simulink model "TxCAN3"  (R2014a)
settings: Solver=ode45  StartTime=0.0  StopTime=10.0  RelTol=1e-3
libraries: simulink x26
settings Model: Creator=10226  LastModifiedBy=10226

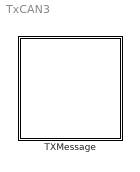
== system TxCAN3 ==
  TXMessage : Subsystem

== system TxCAN3/TXMessage ==
  VCU_AccPedalFault : Ground
  VCU_BMSEmergencyCmd : Ground
  VCU_BMSMainRelayCmd : Ground
  VCU_BrakePedalSts : Ground
  VCU_BrakePedalValue_Reserved : Ground
  VCU_CheckSum : Ground
  VCU_DCDCEnableCmd : Ground
  VCU_DrvControlMode : Ground
  VCU_DrvRequesSpeed : Ground
  VCU_DrvRequestTorque : Ground
  VCU_EA : Subsystem
  VCU_EA_Ter : Terminator
  VCU_ESPTorqReqAvailability : Ground
  VCU_GearLevelPosSts : Ground
  VCU_ParkingReqToEPB : Ground
  VCU_RollingCounter : Ground
  VCU_VehicleSts : Ground
  VCU_Vehicle_Warning : Ground
  wires:
  VCU_ParkingReqToEPB/1 -> VCU_EA/1(VCU_ParkingReqToEPB_in)
  VCU_ESPTorqReqAvailability/1 -> VCU_EA/2(VCU_ESPTorqReqAvailability_in)
  VCU_AccPedalFault/1 -> VCU_EA/3(VCU_AccPedalFault_in)
  VCU_BrakePedalValue_Reserved/1 -> VCU_EA/4(VCU_BrakePedalValue_Reserved_in)
  VCU_CheckSum/1 -> VCU_EA/5(VCU_CheckSum_in)
  VCU_RollingCounter/1 -> VCU_EA/6(VCU_RollingCounter_in)
  VCU_BrakePedalSts/1 -> VCU_EA/7(VCU_BrakePedalSts_in)
  VCU_DCDCEnableCmd/1 -> VCU_EA/8(VCU_DCDCEnableCmd_in)
  VCU_BMSEmergencyCmd/1 -> VCU_EA/9(VCU_BMSEmergencyCmd_in)
  VCU_BMSMainRelayCmd/1 -> VCU_EA/10(VCU_BMSMainRelayCmd_in)
  VCU_GearLevelPosSts/1 -> VCU_EA/11(VCU_GearLevelPosSts_in)
  VCU_VehicleSts/1 -> VCU_EA/12(VCU_VehicleSts_in)
  VCU_Vehicle_Warning/1 -> VCU_EA/13(VCU_Vehicle_Warning_in)
  VCU_DrvControlMode/1 -> VCU_EA/14(VCU_DrvControlMode_in)
  VCU_DrvRequestTorque/1 -> VCU_EA/15(VCU_DrvRequestTorque_in)
  VCU_DrvRequesSpeed/1 -> VCU_EA/16(VCU_DrvRequesSpeed_in)
  VCU_EA/1(output) -> VCU_EA_Ter/1

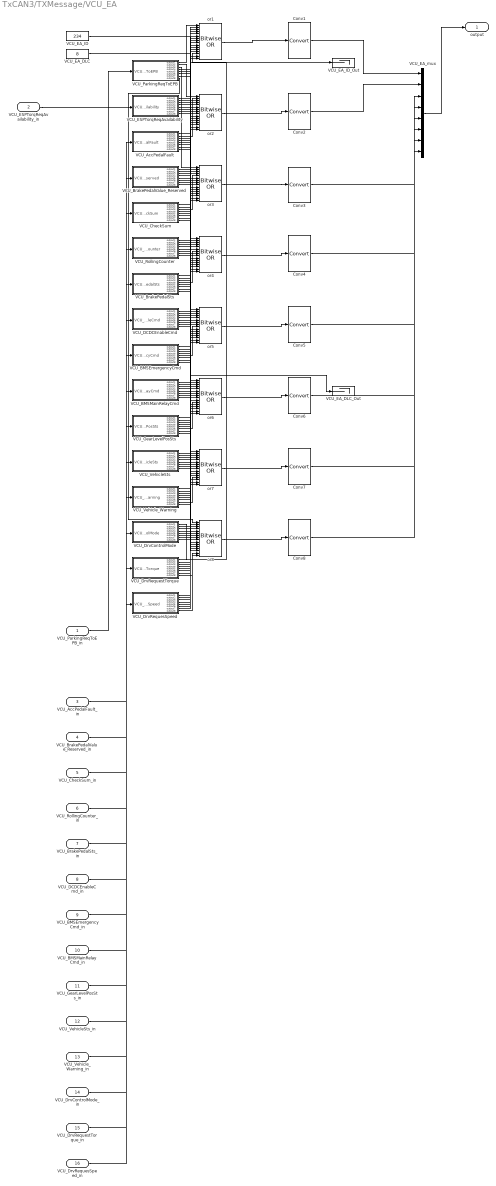
== system TxCAN3/TXMessage/VCU_EA ==
  VCU_ParkingReqToEPB_in : Inport
  VCU_ESPTorqReqAvailability_in : Inport  Port=2
  VCU_AccPedalFault_in : Inport  Port=3
  VCU_BrakePedalValue_Reserved_in : Inport  Port=4
  VCU_CheckSum_in : Inport  Port=5
  VCU_RollingCounter_in : Inport  Port=6
  VCU_BrakePedalSts_in : Inport  Port=7
  VCU_DCDCEnableCmd_in : Inport  Port=8
  VCU_BMSEmergencyCmd_in : Inport  Port=9
  VCU_BMSMainRelayCmd_in : Inport  Port=10
  VCU_GearLevelPosSts_in : Inport  Port=11
  VCU_VehicleSts_in : Inport  Port=12
  VCU_Vehicle_Warning_in : Inport  Port=13
  VCU_DrvControlMode_in : Inport  Port=14
  VCU_DrvRequestTorque_in : Inport  Port=15
  VCU_DrvRequesSpeed_in : Inport  Port=16
  Conv{1..8} (8 alike) : DataTypeConversion
  VCU_AccPedalFault : Subsystem
  VCU_BMSEmergencyCmd : Subsystem
  VCU_BMSMainRelayCmd : Subsystem
  VCU_BrakePedalSts : Subsystem
  VCU_BrakePedalValue_Reserved : Subsystem
  VCU_CheckSum : Subsystem
  VCU_DCDCEnableCmd : Subsystem
  VCU_DrvControlMode : Subsystem
  VCU_DrvRequesSpeed : Subsystem
  VCU_DrvRequestTorque : Subsystem
  VCU_EA_DLC : Constant  Value=8  OutDataTypeStr=uint8
  VCU_EA_DLC_Out : Terminator
  VCU_EA_ID : Constant  Value=234  OutDataTypeStr=single
  VCU_EA_ID_Out : Terminator
  VCU_EA_mux : Mux  Inputs=8
  VCU_ESPTorqReqAvailability : Subsystem
  VCU_GearLevelPosSts : Subsystem
  VCU_ParkingReqToEPB : Subsystem
  VCU_RollingCounter : Subsystem
  VCU_VehicleSts : Subsystem
  VCU_Vehicle_Warning : Subsystem
  or{1..8} (8 alike) : simulink/Logic and Bit Operations/Bitwise Operator  logicop=OR  UseBitMask=off  NumInputPorts=16  BitMask=bin2dec('11011001')  BitMaskRealWorld=Stored Integer
  output : Outport
  wires:
  VCU_EA_mux/1 -> output/1
  VCU_ParkingReqToEPB/1(output1) -> or1/1
  VCU_ParkingReqToEPB/2(output2) -> or2/1
  VCU_ParkingReqToEPB/3(output3) -> or3/1
  VCU_ParkingReqToEPB/4(output4) -> or4/1
  VCU_ParkingReqToEPB/5(output5) -> or5/1
  VCU_ParkingReqToEPB/6(output6) -> or6/1
  VCU_ParkingReqToEPB/7(output7) -> or7/1
  VCU_ParkingReqToEPB/8(output8) -> or8/1
  VCU_ESPTorqReqAvailability/1(output1) -> or1/2
  VCU_ESPTorqReqAvailability/2(output2) -> or2/2
  VCU_ESPTorqReqAvailability/3(output3) -> or3/2
  VCU_ESPTorqReqAvailability/4(output4) -> or4/2
  VCU_ESPTorqReqAvailability/5(output5) -> or5/2
  VCU_ESPTorqReqAvailability/6(output6) -> or6/2
  VCU_ESPTorqReqAvailability/7(output7) -> or7/2
  VCU_ESPTorqReqAvailability/8(output8) -> or8/2
  VCU_AccPedalFault/1(output1) -> or1/3
  VCU_AccPedalFault/2(output2) -> or2/3
  VCU_AccPedalFault/3(output3) -> or3/3
  VCU_AccPedalFault/4(output4) -> or4/3
  VCU_AccPedalFault/5(output5) -> or5/3
  VCU_AccPedalFault/6(output6) -> or6/3
  VCU_AccPedalFault/7(output7) -> or7/3
  VCU_AccPedalFault/8(output8) -> or8/3
  VCU_BrakePedalValue_Reserved/1(output1) -> or1/4
  VCU_BrakePedalValue_Reserved/2(output2) -> or2/4
  VCU_BrakePedalValue_Reserved/3(output3) -> or3/4
  VCU_BrakePedalValue_Reserved/4(output4) -> or4/4
  VCU_BrakePedalValue_Reserved/5(output5) -> or5/4
  VCU_BrakePedalValue_Reserved/6(output6) -> or6/4
  VCU_BrakePedalValue_Reserved/7(output7) -> or7/4
  VCU_BrakePedalValue_Reserved/8(output8) -> or8/4
  VCU_CheckSum/1(output1) -> or1/5
  VCU_CheckSum/2(output2) -> or2/5
  VCU_CheckSum/3(output3) -> or3/5
  VCU_CheckSum/4(output4) -> or4/5
  VCU_CheckSum/5(output5) -> or5/5
  VCU_CheckSum/6(output6) -> or6/5
  VCU_CheckSum/7(output7) -> or7/5
  VCU_CheckSum/8(output8) -> or8/5
  VCU_RollingCounter/1(output1) -> or1/6
  VCU_RollingCounter/2(output2) -> or2/6
  VCU_RollingCounter/3(output3) -> or3/6
  VCU_RollingCounter/4(output4) -> or4/6
  VCU_RollingCounter/5(output5) -> or5/6
  VCU_RollingCounter/6(output6) -> or6/6
  VCU_RollingCounter/7(output7) -> or7/6
  VCU_RollingCounter/8(output8) -> or8/6
  VCU_BrakePedalSts/1(output1) -> or1/7
  VCU_BrakePedalSts/2(output2) -> or2/7
  VCU_BrakePedalSts/3(output3) -> or3/7
  VCU_BrakePedalSts/4(output4) -> or4/7
  VCU_BrakePedalSts/5(output5) -> or5/7
  VCU_BrakePedalSts/6(output6) -> or6/7
  VCU_BrakePedalSts/7(output7) -> or7/7
  VCU_BrakePedalSts/8(output8) -> or8/7
  VCU_DCDCEnableCmd/1(output1) -> or1/8
  VCU_DCDCEnableCmd/2(output2) -> or2/8
  VCU_DCDCEnableCmd/3(output3) -> or3/8
  VCU_DCDCEnableCmd/4(output4) -> or4/8
  VCU_DCDCEnableCmd/5(output5) -> or5/8
  VCU_DCDCEnableCmd/6(output6) -> or6/8
  VCU_DCDCEnableCmd/7(output7) -> or7/8
  VCU_DCDCEnableCmd/8(output8) -> or8/8
  VCU_BMSEmergencyCmd/1(output1) -> or1/9
  VCU_BMSEmergencyCmd/2(output2) -> or2/9
  VCU_BMSEmergencyCmd/3(output3) -> or3/9
  VCU_BMSEmergencyCmd/4(output4) -> or4/9
  VCU_BMSEmergencyCmd/5(output5) -> or5/9
  VCU_BMSEmergencyCmd/6(output6) -> or6/9
  VCU_BMSEmergencyCmd/7(output7) -> or7/9
  VCU_BMSEmergencyCmd/8(output8) -> or8/9
  VCU_BMSMainRelayCmd/1(output1) -> or1/10
  VCU_BMSMainRelayCmd/2(output2) -> or2/10
  VCU_BMSMainRelayCmd/3(output3) -> or3/10
  VCU_BMSMainRelayCmd/4(output4) -> or4/10
  VCU_BMSMainRelayCmd/5(output5) -> or5/10
  VCU_BMSMainRelayCmd/6(output6) -> or6/10
  VCU_BMSMainRelayCmd/7(output7) -> or7/10
  VCU_BMSMainRelayCmd/8(output8) -> or8/10
  VCU_GearLevelPosSts/1(output1) -> or1/11
  VCU_GearLevelPosSts/2(output2) -> or2/11
  VCU_GearLevelPosSts/3(output3) -> or3/11
  VCU_GearLevelPosSts/4(output4) -> or4/11
  VCU_GearLevelPosSts/5(output5) -> or5/11
  VCU_GearLevelPosSts/6(output6) -> or6/11
  VCU_GearLevelPosSts/7(output7) -> or7/11
  VCU_GearLevelPosSts/8(output8) -> or8/11
  VCU_VehicleSts/1(output1) -> or1/12
  VCU_VehicleSts/2(output2) -> or2/12
  VCU_VehicleSts/3(output3) -> or3/12
  VCU_VehicleSts/4(output4) -> or4/12
  VCU_VehicleSts/5(output5) -> or5/12
  VCU_VehicleSts/6(output6) -> or6/12
  VCU_VehicleSts/7(output7) -> or7/12
  VCU_VehicleSts/8(output8) -> or8/12
  VCU_Vehicle_Warning/1(output1) -> or1/13
  VCU_Vehicle_Warning/2(output2) -> or2/13
  VCU_Vehicle_Warning/3(output3) -> or3/13
  VCU_Vehicle_Warning/4(output4) -> or4/13
  VCU_Vehicle_Warning/5(output5) -> or5/13
  VCU_Vehicle_Warning/6(output6) -> or6/13
  VCU_Vehicle_Warning/7(output7) -> or7/13
  VCU_Vehicle_Warning/8(output8) -> or8/13
  VCU_DrvControlMode/1(output1) -> or1/14
  VCU_DrvControlMode/2(output2) -> or2/14
  VCU_DrvControlMode/3(output3) -> or3/14
  VCU_DrvControlMode/4(output4) -> or4/14
  VCU_DrvControlMode/5(output5) -> or5/14
  VCU_DrvControlMode/6(output6) -> or6/14
  VCU_DrvControlMode/7(output7) -> or7/14
  VCU_DrvControlMode/8(output8) -> or8/14
  VCU_DrvRequestTorque/1(output1) -> or1/15
  VCU_DrvRequestTorque/2(output2) -> or2/15
  VCU_DrvRequestTorque/3(output3) -> or3/15
  VCU_DrvRequestTorque/4(output4) -> or4/15
  VCU_DrvRequestTorque/5(output5) -> or5/15
  VCU_DrvRequestTorque/6(output6) -> or6/15
  VCU_DrvRequestTorque/7(output7) -> or7/15
  VCU_DrvRequestTorque/8(output8) -> or8/15
  VCU_DrvRequesSpeed/1(output1) -> or1/16
  VCU_DrvRequesSpeed/2(output2) -> or2/16
  VCU_DrvRequesSpeed/3(output3) -> or3/16
  VCU_DrvRequesSpeed/4(output4) -> or4/16
  VCU_DrvRequesSpeed/5(output5) -> or5/16
  VCU_DrvRequesSpeed/6(output6) -> or6/16
  VCU_DrvRequesSpeed/7(output7) -> or7/16
  VCU_DrvRequesSpeed/8(output8) -> or8/16
  or1/1 -> Conv1/1
  Conv1/1 -> VCU_EA_mux/1
  or2/1 -> Conv2/1
  Conv2/1 -> VCU_EA_mux/2
  or3/1 -> Conv3/1
  Conv3/1 -> VCU_EA_mux/3
  or4/1 -> Conv4/1
  Conv4/1 -> VCU_EA_mux/4
  or5/1 -> Conv5/1
  Conv5/1 -> VCU_EA_mux/5
  or6/1 -> Conv6/1
  Conv6/1 -> VCU_EA_mux/6
  or7/1 -> Conv7/1
  Conv7/1 -> VCU_EA_mux/7
  or8/1 -> Conv8/1
  Conv8/1 -> VCU_EA_mux/8
  VCU_EA_ID/1 -> VCU_EA_ID_Out/1
  VCU_EA_DLC/1 -> VCU_EA_DLC_Out/1
  VCU_ParkingReqToEPB_in/1 -> VCU_ParkingReqToEPB/1(VCU_ParkingReqToEPB)
  VCU_ESPTorqReqAvailability_in/1 -> VCU_ESPTorqReqAvailability/1(VCU_ESPTorqReqAvailability)
  VCU_AccPedalFault_in/1 -> VCU_AccPedalFault/1(VCU_AccPedalFault)
  VCU_BrakePedalValue_Reserved_in/1 -> VCU_BrakePedalValue_Reserved/1(VCU_BrakePedalValue_Reserved)
  VCU_CheckSum_in/1 -> VCU_CheckSum/1(VCU_CheckSum)
  VCU_RollingCounter_in/1 -> VCU_RollingCounter/1(VCU_RollingCounter)
  VCU_BrakePedalSts_in/1 -> VCU_BrakePedalSts/1(VCU_BrakePedalSts)
  VCU_DCDCEnableCmd_in/1 -> VCU_DCDCEnableCmd/1(VCU_DCDCEnableCmd)
  VCU_BMSEmergencyCmd_in/1 -> VCU_BMSEmergencyCmd/1(VCU_BMSEmergencyCmd)
  VCU_BMSMainRelayCmd_in/1 -> VCU_BMSMainRelayCmd/1(VCU_BMSMainRelayCmd)
  VCU_GearLevelPosSts_in/1 -> VCU_GearLevelPosSts/1(VCU_GearLevelPosSts)
  VCU_VehicleSts_in/1 -> VCU_VehicleSts/1(VCU_VehicleSts)
  VCU_Vehicle_Warning_in/1 -> VCU_Vehicle_Warning/1(VCU_Vehicle_Warning)
  VCU_DrvControlMode_in/1 -> VCU_DrvControlMode/1(VCU_DrvControlMode)
  VCU_DrvRequestTorque_in/1 -> VCU_DrvRequestTorque/1(VCU_DrvRequestTorque)
  VCU_DrvRequesSpeed_in/1 -> VCU_DrvRequesSpeed/1(VCU_DrvRequesSpeed)

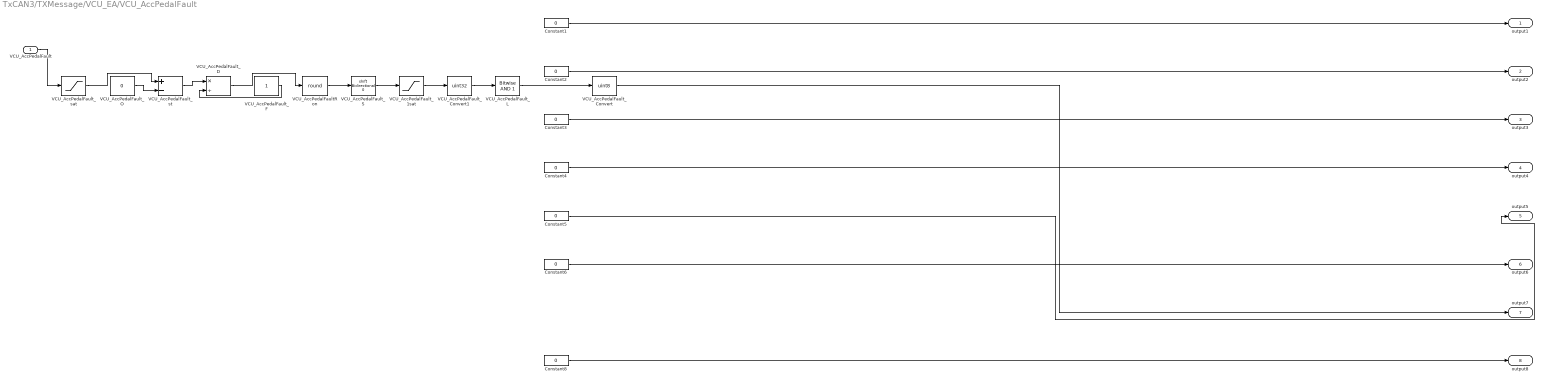
== system TxCAN3/TXMessage/VCU_EA/VCU_AccPedalFault ==
  VCU_AccPedalFault : Inport
  Constant{1..6,8} (7 alike) : Constant  Value=0  OutDataTypeStr=uint8
  VCU_AccPedalFaultRon : Rounding  Operator=round
  VCU_AccPedalFault_1sat : Saturate  UpperLimit=1  LowerLimit=0
  VCU_AccPedalFault_Convert : DataTypeConversion  OutDataTypeStr=uint8
  VCU_AccPedalFault_Convert1 : DataTypeConversion  OutDataTypeStr=uint32
  VCU_AccPedalFault_D : Product  Inputs=*/
  VCU_AccPedalFault_F : Constant  OutDataTypeStr=single
  VCU_AccPedalFault_L : simulink/Logic and Bit Operations/Bitwise Operator  logicop=AND  UseBitMask=on  BitMask=1  BitMaskRealWorld=Stored Integer
  VCU_AccPedalFault_O : Constant  Value=0  OutDataTypeStr=single
  VCU_AccPedalFault_S : ArithShift
  VCU_AccPedalFault_sat : Saturate  UpperLimit=1  LowerLimit=0
  VCU_AccPedalFault_st : Sum  Inputs=+-
  output1 : Outport
  output2 : Outport  Port=2
  output3 : Outport  Port=3
  output4 : Outport  Port=4
  output5 : Outport  Port=5
  output6 : Outport  Port=6
  output7 : Outport  Port=7
  output8 : Outport  Port=8
  wires:
  VCU_AccPedalFault/1 -> VCU_AccPedalFault_sat/1
  VCU_AccPedalFault_sat/1 -> VCU_AccPedalFault_st/1
  VCU_AccPedalFault_O/1 -> VCU_AccPedalFault_st/2
  VCU_AccPedalFault_st/1 -> VCU_AccPedalFault_D/1
  VCU_AccPedalFault_F/1 -> VCU_AccPedalFault_D/2
  VCU_AccPedalFault_D/1 -> VCU_AccPedalFaultRon/1
  VCU_AccPedalFaultRon/1 -> VCU_AccPedalFault_S/1
  VCU_AccPedalFault_S/1 -> VCU_AccPedalFault_1sat/1
  VCU_AccPedalFault_1sat/1 -> VCU_AccPedalFault_Convert1/1
  VCU_AccPedalFault_Convert1/1 -> VCU_AccPedalFault_L/1
  VCU_AccPedalFault_L/1 -> VCU_AccPedalFault_Convert/1
  VCU_AccPedalFault_Convert/1 -> output7/1
  Constant1/1 -> output1/1
  Constant2/1 -> output2/1
  Constant3/1 -> output3/1
  Constant4/1 -> output4/1
  Constant5/1 -> output5/1
  Constant6/1 -> output6/1
  Constant8/1 -> output8/1

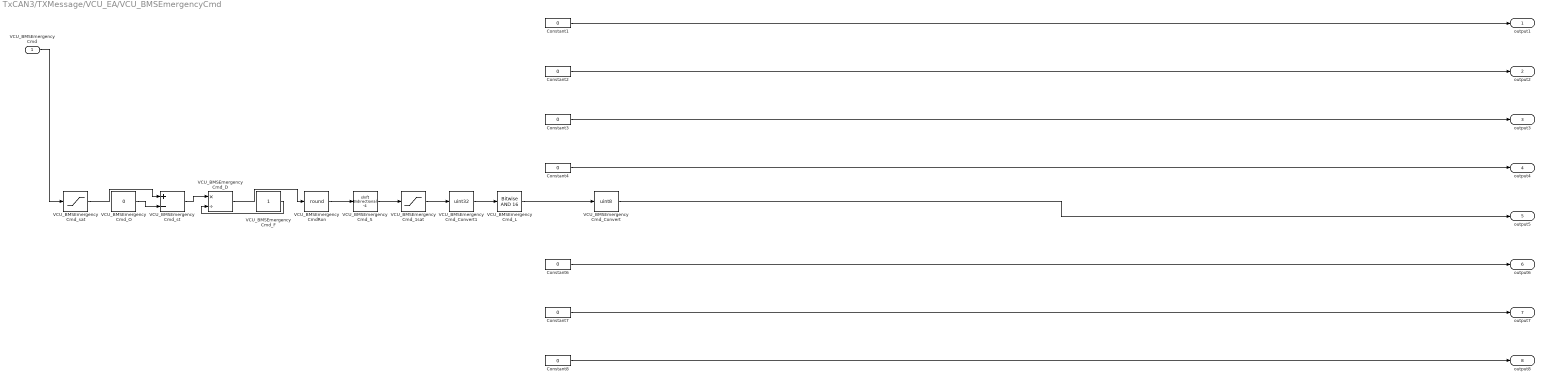
== system TxCAN3/TXMessage/VCU_EA/VCU_BMSEmergencyCmd ==
  VCU_BMSEmergencyCmd : Inport
  Constant{1..4,6..8} (7 alike) : Constant  Value=0  OutDataTypeStr=uint8
  VCU_BMSEmergencyCmdRon : Rounding  Operator=round
  VCU_BMSEmergencyCmd_1sat : Saturate  UpperLimit=16  LowerLimit=0
  VCU_BMSEmergencyCmd_Convert : DataTypeConversion  OutDataTypeStr=uint8
  VCU_BMSEmergencyCmd_Convert1 : DataTypeConversion  OutDataTypeStr=uint32
  VCU_BMSEmergencyCmd_D : Product  Inputs=*/
  VCU_BMSEmergencyCmd_F : Constant  OutDataTypeStr=single
  VCU_BMSEmergencyCmd_L : simulink/Logic and Bit Operations/Bitwise Operator  logicop=AND  UseBitMask=on  BitMask=16  BitMaskRealWorld=Stored Integer
  VCU_BMSEmergencyCmd_O : Constant  Value=0  OutDataTypeStr=single
  VCU_BMSEmergencyCmd_S : ArithShift  BitShiftNumber=-4
  VCU_BMSEmergencyCmd_sat : Saturate  UpperLimit=1  LowerLimit=0
  VCU_BMSEmergencyCmd_st : Sum  Inputs=+-
  output1 : Outport
  output2 : Outport  Port=2
  output3 : Outport  Port=3
  output4 : Outport  Port=4
  output5 : Outport  Port=5
  output6 : Outport  Port=6
  output7 : Outport  Port=7
  output8 : Outport  Port=8
  wires:
  VCU_BMSEmergencyCmd/1 -> VCU_BMSEmergencyCmd_sat/1
  VCU_BMSEmergencyCmd_sat/1 -> VCU_BMSEmergencyCmd_st/1
  VCU_BMSEmergencyCmd_O/1 -> VCU_BMSEmergencyCmd_st/2
  VCU_BMSEmergencyCmd_st/1 -> VCU_BMSEmergencyCmd_D/1
  VCU_BMSEmergencyCmd_F/1 -> VCU_BMSEmergencyCmd_D/2
  VCU_BMSEmergencyCmd_D/1 -> VCU_BMSEmergencyCmdRon/1
  VCU_BMSEmergencyCmdRon/1 -> VCU_BMSEmergencyCmd_S/1
  VCU_BMSEmergencyCmd_S/1 -> VCU_BMSEmergencyCmd_1sat/1
  VCU_BMSEmergencyCmd_1sat/1 -> VCU_BMSEmergencyCmd_Convert1/1
  VCU_BMSEmergencyCmd_Convert1/1 -> VCU_BMSEmergencyCmd_L/1
  VCU_BMSEmergencyCmd_L/1 -> VCU_BMSEmergencyCmd_Convert/1
  VCU_BMSEmergencyCmd_Convert/1 -> output5/1
  Constant1/1 -> output1/1
  Constant2/1 -> output2/1
  Constant3/1 -> output3/1
  Constant4/1 -> output4/1
  Constant6/1 -> output6/1
  Constant7/1 -> output7/1
  Constant8/1 -> output8/1

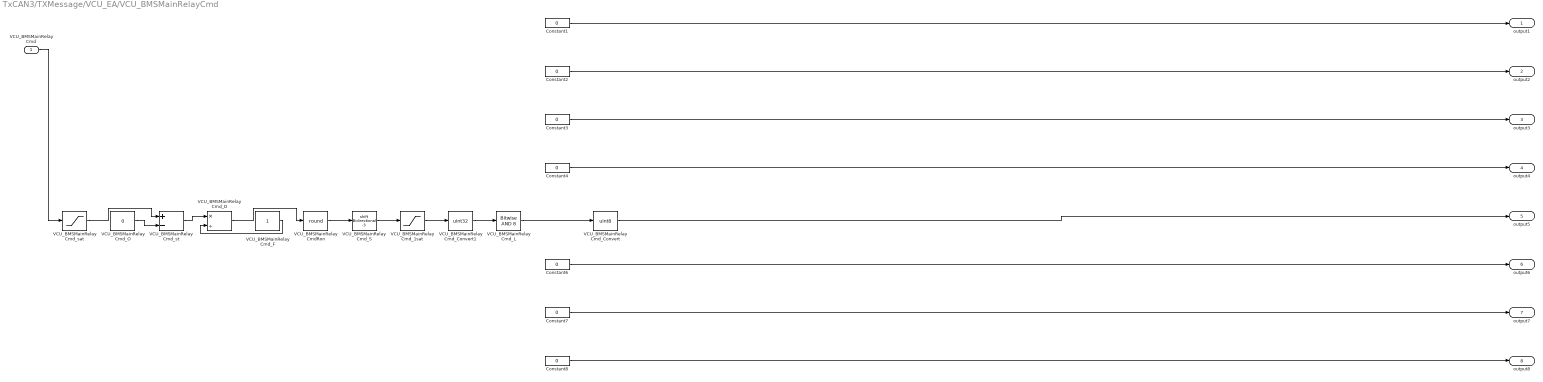
== system TxCAN3/TXMessage/VCU_EA/VCU_BMSMainRelayCmd ==
  VCU_BMSMainRelayCmd : Inport
  Constant{1..4,6..8} (7 alike) : Constant  Value=0  OutDataTypeStr=uint8
  VCU_BMSMainRelayCmdRon : Rounding  Operator=round
  VCU_BMSMainRelayCmd_1sat : Saturate  UpperLimit=8  LowerLimit=0
  VCU_BMSMainRelayCmd_Convert : DataTypeConversion  OutDataTypeStr=uint8
  VCU_BMSMainRelayCmd_Convert1 : DataTypeConversion  OutDataTypeStr=uint32
  VCU_BMSMainRelayCmd_D : Product  Inputs=*/
  VCU_BMSMainRelayCmd_F : Constant  OutDataTypeStr=single
  VCU_BMSMainRelayCmd_L : simulink/Logic and Bit Operations/Bitwise Operator  logicop=AND  UseBitMask=on  BitMask=8  BitMaskRealWorld=Stored Integer
  VCU_BMSMainRelayCmd_O : Constant  Value=0  OutDataTypeStr=single
  VCU_BMSMainRelayCmd_S : ArithShift  BitShiftNumber=-3
  VCU_BMSMainRelayCmd_sat : Saturate  UpperLimit=1  LowerLimit=0
  VCU_BMSMainRelayCmd_st : Sum  Inputs=+-
  output1 : Outport
  output2 : Outport  Port=2
  output3 : Outport  Port=3
  output4 : Outport  Port=4
  output5 : Outport  Port=5
  output6 : Outport  Port=6
  output7 : Outport  Port=7
  output8 : Outport  Port=8
  wires:
  VCU_BMSMainRelayCmd/1 -> VCU_BMSMainRelayCmd_sat/1
  VCU_BMSMainRelayCmd_sat/1 -> VCU_BMSMainRelayCmd_st/1
  VCU_BMSMainRelayCmd_O/1 -> VCU_BMSMainRelayCmd_st/2
  VCU_BMSMainRelayCmd_st/1 -> VCU_BMSMainRelayCmd_D/1
  VCU_BMSMainRelayCmd_F/1 -> VCU_BMSMainRelayCmd_D/2
  VCU_BMSMainRelayCmd_D/1 -> VCU_BMSMainRelayCmdRon/1
  VCU_BMSMainRelayCmdRon/1 -> VCU_BMSMainRelayCmd_S/1
  VCU_BMSMainRelayCmd_S/1 -> VCU_BMSMainRelayCmd_1sat/1
  VCU_BMSMainRelayCmd_1sat/1 -> VCU_BMSMainRelayCmd_Convert1/1
  VCU_BMSMainRelayCmd_Convert1/1 -> VCU_BMSMainRelayCmd_L/1
  VCU_BMSMainRelayCmd_L/1 -> VCU_BMSMainRelayCmd_Convert/1
  VCU_BMSMainRelayCmd_Convert/1 -> output5/1
  Constant1/1 -> output1/1
  Constant2/1 -> output2/1
  Constant3/1 -> output3/1
  Constant4/1 -> output4/1
  Constant6/1 -> output6/1
  Constant7/1 -> output7/1
  Constant8/1 -> output8/1

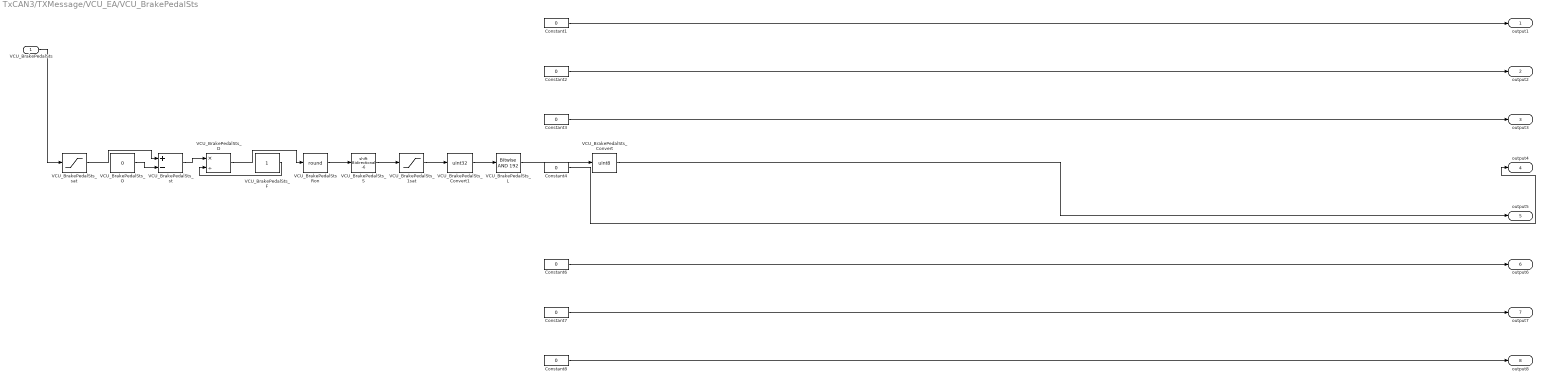
== system TxCAN3/TXMessage/VCU_EA/VCU_BrakePedalSts ==
  VCU_BrakePedalSts : Inport
  Constant{1..4,6..8} (7 alike) : Constant  Value=0  OutDataTypeStr=uint8
  VCU_BrakePedalStsRon : Rounding  Operator=round
  VCU_BrakePedalSts_1sat : Saturate  UpperLimit=192  LowerLimit=0
  VCU_BrakePedalSts_Convert : DataTypeConversion  OutDataTypeStr=uint8
  VCU_BrakePedalSts_Convert1 : DataTypeConversion  OutDataTypeStr=uint32
  VCU_BrakePedalSts_D : Product  Inputs=*/
  VCU_BrakePedalSts_F : Constant  OutDataTypeStr=single
  VCU_BrakePedalSts_L : simulink/Logic and Bit Operations/Bitwise Operator  logicop=AND  UseBitMask=on  BitMask=192  BitMaskRealWorld=Stored Integer
  VCU_BrakePedalSts_O : Constant  Value=0  OutDataTypeStr=single
  VCU_BrakePedalSts_S : ArithShift  BitShiftNumber=-6
  VCU_BrakePedalSts_sat : Saturate  UpperLimit=3  LowerLimit=0
  VCU_BrakePedalSts_st : Sum  Inputs=+-
  output1 : Outport
  output2 : Outport  Port=2
  output3 : Outport  Port=3
  output4 : Outport  Port=4
  output5 : Outport  Port=5
  output6 : Outport  Port=6
  output7 : Outport  Port=7
  output8 : Outport  Port=8
  wires:
  VCU_BrakePedalSts/1 -> VCU_BrakePedalSts_sat/1
  VCU_BrakePedalSts_sat/1 -> VCU_BrakePedalSts_st/1
  VCU_BrakePedalSts_O/1 -> VCU_BrakePedalSts_st/2
  VCU_BrakePedalSts_st/1 -> VCU_BrakePedalSts_D/1
  VCU_BrakePedalSts_F/1 -> VCU_BrakePedalSts_D/2
  VCU_BrakePedalSts_D/1 -> VCU_BrakePedalStsRon/1
  VCU_BrakePedalStsRon/1 -> VCU_BrakePedalSts_S/1
  VCU_BrakePedalSts_S/1 -> VCU_BrakePedalSts_1sat/1
  VCU_BrakePedalSts_1sat/1 -> VCU_BrakePedalSts_Convert1/1
  VCU_BrakePedalSts_Convert1/1 -> VCU_BrakePedalSts_L/1
  VCU_BrakePedalSts_L/1 -> VCU_BrakePedalSts_Convert/1
  VCU_BrakePedalSts_Convert/1 -> output5/1
  Constant1/1 -> output1/1
  Constant2/1 -> output2/1
  Constant3/1 -> output3/1
  Constant4/1 -> output4/1
  Constant6/1 -> output6/1
  Constant7/1 -> output7/1
  Constant8/1 -> output8/1

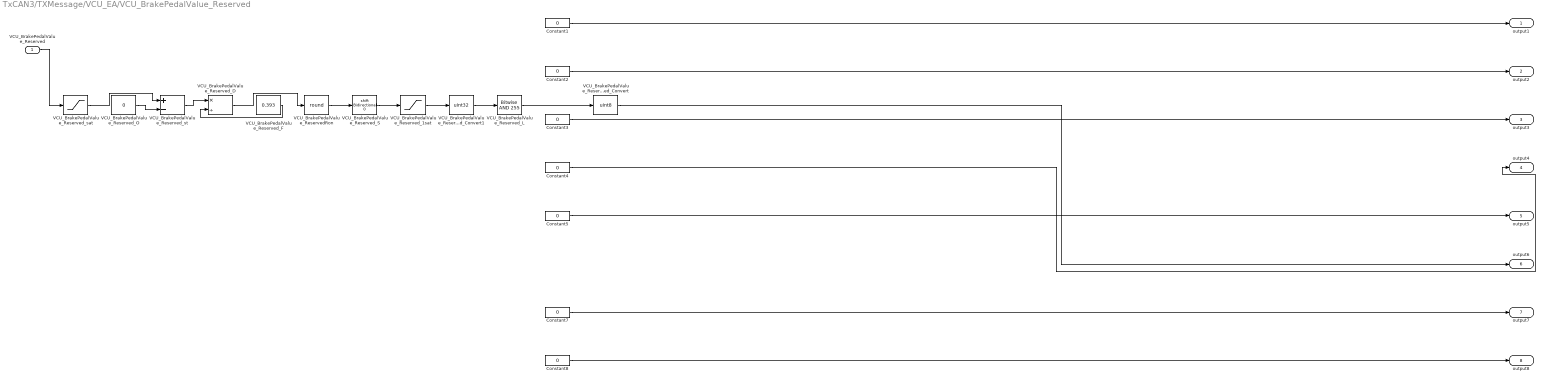
== system TxCAN3/TXMessage/VCU_EA/VCU_BrakePedalValue_Reserved ==
  VCU_BrakePedalValue_Reserved : Inport
  Constant{1..5,7..8} (7 alike) : Constant  Value=0  OutDataTypeStr=uint8
  VCU_BrakePedalValue_ReservedRon : Rounding  Operator=round
  VCU_BrakePedalValue_Reserved_1sat : Saturate  UpperLimit=255  LowerLimit=0
  VCU_BrakePedalValue_Reserved_Convert : DataTypeConversion  OutDataTypeStr=uint8
  VCU_BrakePedalValue_Reserved_Convert1 : DataTypeConversion  OutDataTypeStr=uint32
  VCU_BrakePedalValue_Reserved_D : Product  Inputs=*/
  VCU_BrakePedalValue_Reserved_F : Constant  Value=0.393  OutDataTypeStr=single
  VCU_BrakePedalValue_Reserved_L : simulink/Logic and Bit Operations/Bitwise Operator  logicop=AND  UseBitMask=on  BitMask=255  BitMaskRealWorld=Stored Integer
  VCU_BrakePedalValue_Reserved_O : Constant  Value=0  OutDataTypeStr=single
  VCU_BrakePedalValue_Reserved_S : ArithShift
  VCU_BrakePedalValue_Reserved_sat : Saturate  UpperLimit=100  LowerLimit=0
  VCU_BrakePedalValue_Reserved_st : Sum  Inputs=+-
  output1 : Outport
  output2 : Outport  Port=2
  output3 : Outport  Port=3
  output4 : Outport  Port=4
  output5 : Outport  Port=5
  output6 : Outport  Port=6
  output7 : Outport  Port=7
  output8 : Outport  Port=8
  wires:
  VCU_BrakePedalValue_Reserved/1 -> VCU_BrakePedalValue_Reserved_sat/1
  VCU_BrakePedalValue_Reserved_sat/1 -> VCU_BrakePedalValue_Reserved_st/1
  VCU_BrakePedalValue_Reserved_O/1 -> VCU_BrakePedalValue_Reserved_st/2
  VCU_BrakePedalValue_Reserved_st/1 -> VCU_BrakePedalValue_Reserved_D/1
  VCU_BrakePedalValue_Reserved_F/1 -> VCU_BrakePedalValue_Reserved_D/2
  VCU_BrakePedalValue_Reserved_D/1 -> VCU_BrakePedalValue_ReservedRon/1
  VCU_BrakePedalValue_ReservedRon/1 -> VCU_BrakePedalValue_Reserved_S/1
  VCU_BrakePedalValue_Reserved_S/1 -> VCU_BrakePedalValue_Reserved_1sat/1
  VCU_BrakePedalValue_Reserved_1sat/1 -> VCU_BrakePedalValue_Reserved_Convert1/1
  VCU_BrakePedalValue_Reserved_Convert1/1 -> VCU_BrakePedalValue_Reserved_L/1
  VCU_BrakePedalValue_Reserved_L/1 -> VCU_BrakePedalValue_Reserved_Convert/1
  VCU_BrakePedalValue_Reserved_Convert/1 -> output6/1
  Constant1/1 -> output1/1
  Constant2/1 -> output2/1
  Constant3/1 -> output3/1
  Constant4/1 -> output4/1
  Constant5/1 -> output5/1
  Constant7/1 -> output7/1
  Constant8/1 -> output8/1

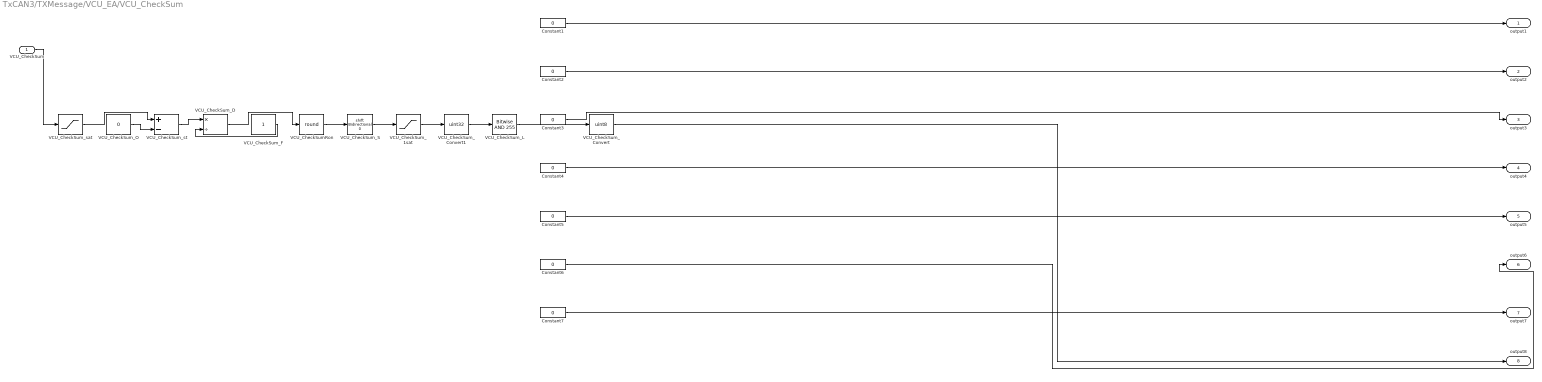
== system TxCAN3/TXMessage/VCU_EA/VCU_CheckSum ==
  VCU_CheckSum : Inport
  Constant{1..7} (7 alike) : Constant  Value=0  OutDataTypeStr=uint8
  VCU_CheckSumRon : Rounding  Operator=round
  VCU_CheckSum_1sat : Saturate  UpperLimit=255  LowerLimit=0
  VCU_CheckSum_Convert : DataTypeConversion  OutDataTypeStr=uint8
  VCU_CheckSum_Convert1 : DataTypeConversion  OutDataTypeStr=uint32
  VCU_CheckSum_D : Product  Inputs=*/
  VCU_CheckSum_F : Constant  OutDataTypeStr=single
  VCU_CheckSum_L : simulink/Logic and Bit Operations/Bitwise Operator  logicop=AND  UseBitMask=on  BitMask=255  BitMaskRealWorld=Stored Integer
  VCU_CheckSum_O : Constant  Value=0  OutDataTypeStr=single
  VCU_CheckSum_S : ArithShift
  VCU_CheckSum_sat : Saturate  UpperLimit=255  LowerLimit=0
  VCU_CheckSum_st : Sum  Inputs=+-
  output1 : Outport
  output2 : Outport  Port=2
  output3 : Outport  Port=3
  output4 : Outport  Port=4
  output5 : Outport  Port=5
  output6 : Outport  Port=6
  output7 : Outport  Port=7
  output8 : Outport  Port=8
  wires:
  VCU_CheckSum/1 -> VCU_CheckSum_sat/1
  VCU_CheckSum_sat/1 -> VCU_CheckSum_st/1
  VCU_CheckSum_O/1 -> VCU_CheckSum_st/2
  VCU_CheckSum_st/1 -> VCU_CheckSum_D/1
  VCU_CheckSum_F/1 -> VCU_CheckSum_D/2
  VCU_CheckSum_D/1 -> VCU_CheckSumRon/1
  VCU_CheckSumRon/1 -> VCU_CheckSum_S/1
  VCU_CheckSum_S/1 -> VCU_CheckSum_1sat/1
  VCU_CheckSum_1sat/1 -> VCU_CheckSum_Convert1/1
  VCU_CheckSum_Convert1/1 -> VCU_CheckSum_L/1
  VCU_CheckSum_L/1 -> VCU_CheckSum_Convert/1
  VCU_CheckSum_Convert/1 -> output8/1
  Constant1/1 -> output1/1
  Constant2/1 -> output2/1
  Constant3/1 -> output3/1
  Constant4/1 -> output4/1
  Constant5/1 -> output5/1
  Constant6/1 -> output6/1
  Constant7/1 -> output7/1

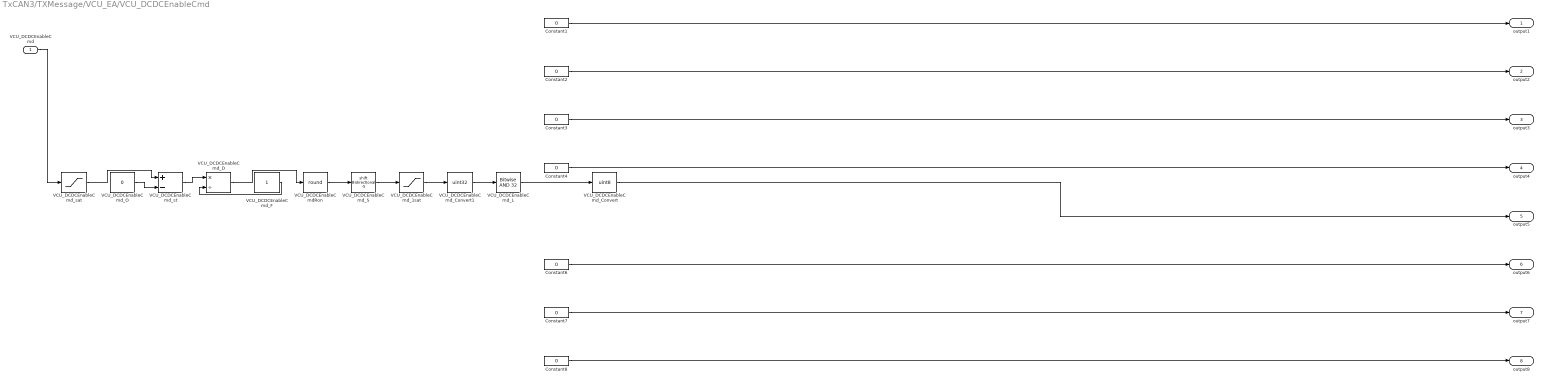
== system TxCAN3/TXMessage/VCU_EA/VCU_DCDCEnableCmd ==
  VCU_DCDCEnableCmd : Inport
  Constant{1..4,6..8} (7 alike) : Constant  Value=0  OutDataTypeStr=uint8
  VCU_DCDCEnableCmdRon : Rounding  Operator=round
  VCU_DCDCEnableCmd_1sat : Saturate  UpperLimit=32  LowerLimit=0
  VCU_DCDCEnableCmd_Convert : DataTypeConversion  OutDataTypeStr=uint8
  VCU_DCDCEnableCmd_Convert1 : DataTypeConversion  OutDataTypeStr=uint32
  VCU_DCDCEnableCmd_D : Product  Inputs=*/
  VCU_DCDCEnableCmd_F : Constant  OutDataTypeStr=single
  VCU_DCDCEnableCmd_L : simulink/Logic and Bit Operations/Bitwise Operator  logicop=AND  UseBitMask=on  BitMask=32  BitMaskRealWorld=Stored Integer
  VCU_DCDCEnableCmd_O : Constant  Value=0  OutDataTypeStr=single
  VCU_DCDCEnableCmd_S : ArithShift  BitShiftNumber=-5
  VCU_DCDCEnableCmd_sat : Saturate  UpperLimit=1  LowerLimit=0
  VCU_DCDCEnableCmd_st : Sum  Inputs=+-
  output1 : Outport
  output2 : Outport  Port=2
  output3 : Outport  Port=3
  output4 : Outport  Port=4
  output5 : Outport  Port=5
  output6 : Outport  Port=6
  output7 : Outport  Port=7
  output8 : Outport  Port=8
  wires:
  VCU_DCDCEnableCmd/1 -> VCU_DCDCEnableCmd_sat/1
  VCU_DCDCEnableCmd_sat/1 -> VCU_DCDCEnableCmd_st/1
  VCU_DCDCEnableCmd_O/1 -> VCU_DCDCEnableCmd_st/2
  VCU_DCDCEnableCmd_st/1 -> VCU_DCDCEnableCmd_D/1
  VCU_DCDCEnableCmd_F/1 -> VCU_DCDCEnableCmd_D/2
  VCU_DCDCEnableCmd_D/1 -> VCU_DCDCEnableCmdRon/1
  VCU_DCDCEnableCmdRon/1 -> VCU_DCDCEnableCmd_S/1
  VCU_DCDCEnableCmd_S/1 -> VCU_DCDCEnableCmd_1sat/1
  VCU_DCDCEnableCmd_1sat/1 -> VCU_DCDCEnableCmd_Convert1/1
  VCU_DCDCEnableCmd_Convert1/1 -> VCU_DCDCEnableCmd_L/1
  VCU_DCDCEnableCmd_L/1 -> VCU_DCDCEnableCmd_Convert/1
  VCU_DCDCEnableCmd_Convert/1 -> output5/1
  Constant1/1 -> output1/1
  Constant2/1 -> output2/1
  Constant3/1 -> output3/1
  Constant4/1 -> output4/1
  Constant6/1 -> output6/1
  Constant7/1 -> output7/1
  Constant8/1 -> output8/1

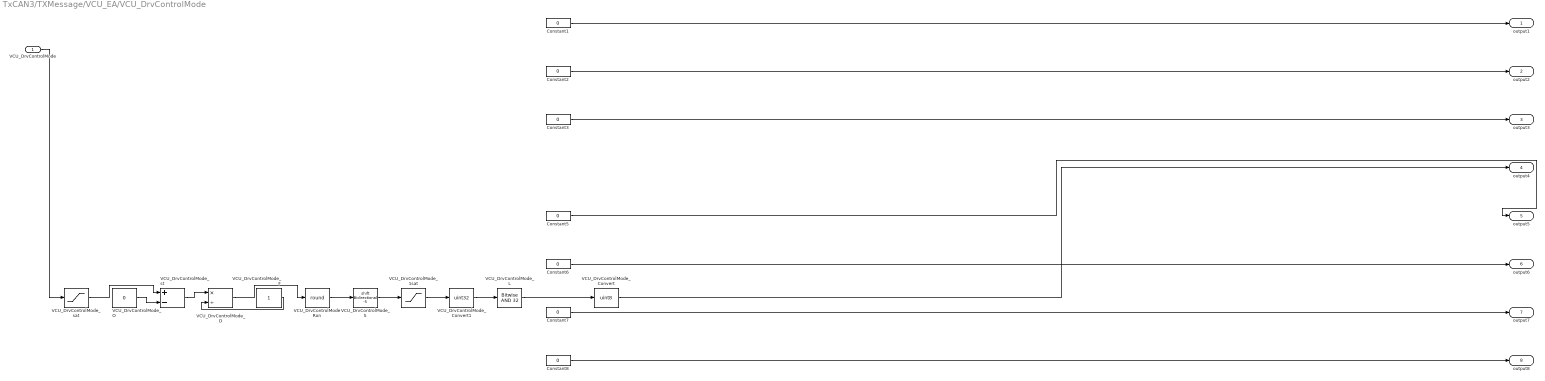
== system TxCAN3/TXMessage/VCU_EA/VCU_DrvControlMode ==
  VCU_DrvControlMode : Inport
  Constant{1..3,5..8} (7 alike) : Constant  Value=0  OutDataTypeStr=uint8
  VCU_DrvControlModeRon : Rounding  Operator=round
  VCU_DrvControlMode_1sat : Saturate  UpperLimit=32  LowerLimit=0
  VCU_DrvControlMode_Convert : DataTypeConversion  OutDataTypeStr=uint8
  VCU_DrvControlMode_Convert1 : DataTypeConversion  OutDataTypeStr=uint32
  VCU_DrvControlMode_D : Product  Inputs=*/
  VCU_DrvControlMode_F : Constant  OutDataTypeStr=single
  VCU_DrvControlMode_L : simulink/Logic and Bit Operations/Bitwise Operator  logicop=AND  UseBitMask=on  BitMask=32  BitMaskRealWorld=Stored Integer
  VCU_DrvControlMode_O : Constant  Value=0  OutDataTypeStr=single
  VCU_DrvControlMode_S : ArithShift  BitShiftNumber=-5
  VCU_DrvControlMode_sat : Saturate  UpperLimit=1  LowerLimit=0
  VCU_DrvControlMode_st : Sum  Inputs=+-
  output1 : Outport
  output2 : Outport  Port=2
  output3 : Outport  Port=3
  output4 : Outport  Port=4
  output5 : Outport  Port=5
  output6 : Outport  Port=6
  output7 : Outport  Port=7
  output8 : Outport  Port=8
  wires:
  VCU_DrvControlMode/1 -> VCU_DrvControlMode_sat/1
  VCU_DrvControlMode_sat/1 -> VCU_DrvControlMode_st/1
  VCU_DrvControlMode_O/1 -> VCU_DrvControlMode_st/2
  VCU_DrvControlMode_st/1 -> VCU_DrvControlMode_D/1
  VCU_DrvControlMode_F/1 -> VCU_DrvControlMode_D/2
  VCU_DrvControlMode_D/1 -> VCU_DrvControlModeRon/1
  VCU_DrvControlModeRon/1 -> VCU_DrvControlMode_S/1
  VCU_DrvControlMode_S/1 -> VCU_DrvControlMode_1sat/1
  VCU_DrvControlMode_1sat/1 -> VCU_DrvControlMode_Convert1/1
  VCU_DrvControlMode_Convert1/1 -> VCU_DrvControlMode_L/1
  VCU_DrvControlMode_L/1 -> VCU_DrvControlMode_Convert/1
  VCU_DrvControlMode_Convert/1 -> output4/1
  Constant1/1 -> output1/1
  Constant2/1 -> output2/1
  Constant3/1 -> output3/1
  Constant5/1 -> output5/1
  Constant6/1 -> output6/1
  Constant7/1 -> output7/1
  Constant8/1 -> output8/1

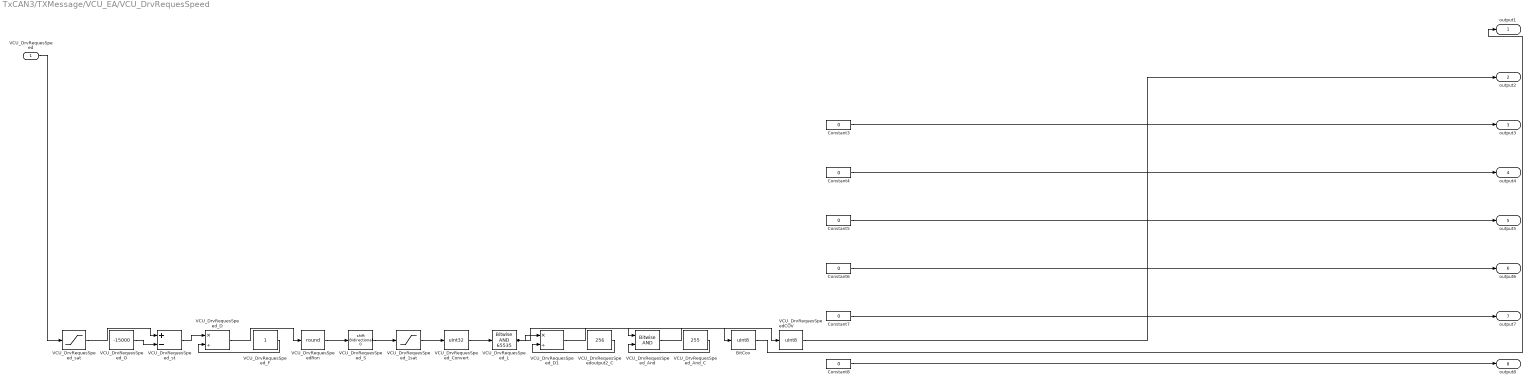
== system TxCAN3/TXMessage/VCU_EA/VCU_DrvRequesSpeed ==
  VCU_DrvRequesSpeed : Inport
  BitCov : DataTypeConversion  OutDataTypeStr=uint8
  Constant{3..8} (6 alike) : Constant  Value=0  OutDataTypeStr=uint8
  VCU_DrvRequesSpeedCOV : DataTypeConversion  OutDataTypeStr=uint8
  VCU_DrvRequesSpeedRon : Rounding  Operator=round
  VCU_DrvRequesSpeed_1sat : Saturate  UpperLimit=65535  LowerLimit=0
  VCU_DrvRequesSpeed_And : simulink/Logic and Bit Operations/Bitwise Operator  logicop=AND  UseBitMask=off  NumInputPorts=2  BitMask=bin2dec('11011001')  BitMaskRealWorld=Stored Integer
  VCU_DrvRequesSpeed_And_C : Constant  Value=255  OutDataTypeStr=uint32
  VCU_DrvRequesSpeed_Convert : DataTypeConversion  OutDataTypeStr=uint32
  VCU_DrvRequesSpeed_D : Product  Inputs=*/
  VCU_DrvRequesSpeed_D1 : Product  Inputs=*/
  VCU_DrvRequesSpeed_F : Constant  OutDataTypeStr=single
  VCU_DrvRequesSpeed_L : simulink/Logic and Bit Operations/Bitwise Operator  logicop=AND  UseBitMask=on  BitMask=65535  BitMaskRealWorld=Stored Integer
  VCU_DrvRequesSpeed_O : Constant  Value=-15000  OutDataTypeStr=single
  VCU_DrvRequesSpeed_S : ArithShift
  VCU_DrvRequesSpeed_sat : Saturate  UpperLimit=15000  LowerLimit=-15000
  VCU_DrvRequesSpeed_st : Sum  Inputs=+-
  VCU_DrvRequesSpeedoutput2_C : Constant  Value=256
  output1 : Outport
  output2 : Outport  Port=2
  output3 : Outport  Port=3
  output4 : Outport  Port=4
  output5 : Outport  Port=5
  output6 : Outport  Port=6
  output7 : Outport  Port=7
  output8 : Outport  Port=8
  wires:
  VCU_DrvRequesSpeed/1 -> VCU_DrvRequesSpeed_sat/1
  VCU_DrvRequesSpeed_sat/1 -> VCU_DrvRequesSpeed_st/1
  VCU_DrvRequesSpeed_O/1 -> VCU_DrvRequesSpeed_st/2
  VCU_DrvRequesSpeed_st/1 -> VCU_DrvRequesSpeed_D/1
  VCU_DrvRequesSpeed_F/1 -> VCU_DrvRequesSpeed_D/2
  VCU_DrvRequesSpeed_D/1 -> VCU_DrvRequesSpeedRon/1
  VCU_DrvRequesSpeedRon/1 -> VCU_DrvRequesSpeed_S/1
  VCU_DrvRequesSpeed_S/1 -> VCU_DrvRequesSpeed_1sat/1
  VCU_DrvRequesSpeed_1sat/1 -> VCU_DrvRequesSpeed_Convert/1
  VCU_DrvRequesSpeed_Convert/1 -> VCU_DrvRequesSpeed_L/1
  VCU_DrvRequesSpeed_L/1 -> VCU_DrvRequesSpeed_D1/1, VCU_DrvRequesSpeed_And/1
  VCU_DrvRequesSpeedoutput2_C/1 -> VCU_DrvRequesSpeed_D1/2
  VCU_DrvRequesSpeed_D1/1 -> VCU_DrvRequesSpeedCOV/1
  VCU_DrvRequesSpeedCOV/1 -> output2/1
  VCU_DrvRequesSpeed_And_C/1 -> VCU_DrvRequesSpeed_And/2
  VCU_DrvRequesSpeed_And/1 -> BitCov/1
  BitCov/1 -> output1/1
  Constant3/1 -> output3/1
  Constant4/1 -> output4/1
  Constant5/1 -> output5/1
  Constant6/1 -> output6/1
  Constant7/1 -> output7/1
  Constant8/1 -> output8/1

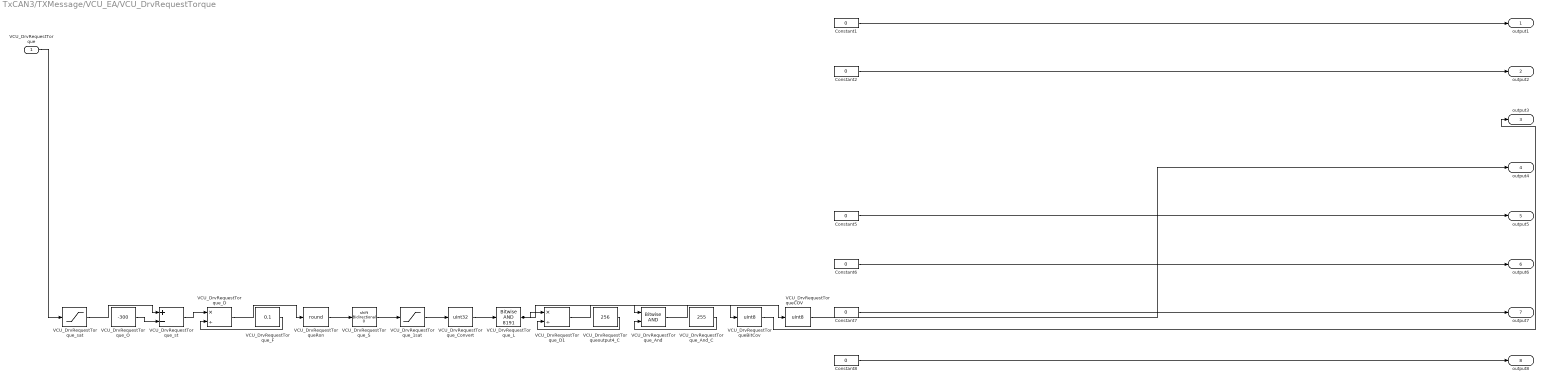
== system TxCAN3/TXMessage/VCU_EA/VCU_DrvRequestTorque ==
  VCU_DrvRequestTorque : Inport
  Constant{1..2,5..8} (6 alike) : Constant  Value=0  OutDataTypeStr=uint8
  VCU_DrvRequestTorqueBitCov : DataTypeConversion  OutDataTypeStr=uint8
  VCU_DrvRequestTorqueCOV : DataTypeConversion  OutDataTypeStr=uint8
  VCU_DrvRequestTorqueRon : Rounding  Operator=round
  VCU_DrvRequestTorque_1sat : Saturate  UpperLimit=8191  LowerLimit=0
  VCU_DrvRequestTorque_And : simulink/Logic and Bit Operations/Bitwise Operator  logicop=AND  UseBitMask=off  NumInputPorts=2  BitMask=bin2dec('11011001')  BitMaskRealWorld=Stored Integer
  VCU_DrvRequestTorque_And_C : Constant  Value=255  OutDataTypeStr=uint32
  VCU_DrvRequestTorque_Convert : DataTypeConversion  OutDataTypeStr=uint32
  VCU_DrvRequestTorque_D : Product  Inputs=*/
  VCU_DrvRequestTorque_D1 : Product  Inputs=*/
  VCU_DrvRequestTorque_F : Constant  Value=0.1  OutDataTypeStr=single
  VCU_DrvRequestTorque_L : simulink/Logic and Bit Operations/Bitwise Operator  logicop=AND  UseBitMask=on  BitMask=8191  BitMaskRealWorld=Stored Integer
  VCU_DrvRequestTorque_O : Constant  Value=-300  OutDataTypeStr=single
  VCU_DrvRequestTorque_S : ArithShift
  VCU_DrvRequestTorque_sat : Saturate  UpperLimit=300  LowerLimit=-300
  VCU_DrvRequestTorque_st : Sum  Inputs=+-
  VCU_DrvRequestTorqueoutput4_C : Constant  Value=256
  output1 : Outport
  output2 : Outport  Port=2
  output3 : Outport  Port=3
  output4 : Outport  Port=4
  output5 : Outport  Port=5
  output6 : Outport  Port=6
  output7 : Outport  Port=7
  output8 : Outport  Port=8
  wires:
  VCU_DrvRequestTorque/1 -> VCU_DrvRequestTorque_sat/1
  VCU_DrvRequestTorque_sat/1 -> VCU_DrvRequestTorque_st/1
  VCU_DrvRequestTorque_O/1 -> VCU_DrvRequestTorque_st/2
  VCU_DrvRequestTorque_st/1 -> VCU_DrvRequestTorque_D/1
  VCU_DrvRequestTorque_F/1 -> VCU_DrvRequestTorque_D/2
  VCU_DrvRequestTorque_D/1 -> VCU_DrvRequestTorqueRon/1
  VCU_DrvRequestTorqueRon/1 -> VCU_DrvRequestTorque_S/1
  VCU_DrvRequestTorque_S/1 -> VCU_DrvRequestTorque_1sat/1
  VCU_DrvRequestTorque_1sat/1 -> VCU_DrvRequestTorque_Convert/1
  VCU_DrvRequestTorque_Convert/1 -> VCU_DrvRequestTorque_L/1
  VCU_DrvRequestTorque_L/1 -> VCU_DrvRequestTorque_D1/1, VCU_DrvRequestTorque_And/1
  VCU_DrvRequestTorqueoutput4_C/1 -> VCU_DrvRequestTorque_D1/2
  VCU_DrvRequestTorque_D1/1 -> VCU_DrvRequestTorqueCOV/1
  VCU_DrvRequestTorqueCOV/1 -> output4/1
  VCU_DrvRequestTorque_And_C/1 -> VCU_DrvRequestTorque_And/2
  VCU_DrvRequestTorque_And/1 -> VCU_DrvRequestTorqueBitCov/1
  VCU_DrvRequestTorqueBitCov/1 -> output3/1
  Constant1/1 -> output1/1
  Constant2/1 -> output2/1
  Constant5/1 -> output5/1
  Constant6/1 -> output6/1
  Constant7/1 -> output7/1
  Constant8/1 -> output8/1

== system TxCAN3/TXMessage/VCU_EA/VCU_ESPTorqReqAvailability ==
  VCU_ESPTorqReqAvailability : Inport
  Constant{1..6,8} (7 alike) : Constant  Value=0  OutDataTypeStr=uint8
  VCU_ESPTorqReqAvailabilityRon : Rounding  Operator=round
  VCU_ESPTorqReqAvailability_1sat : Saturate  UpperLimit=2  LowerLimit=0
  VCU_ESPTorqReqAvailability_Convert : DataTypeConversion  OutDataTypeStr=uint8
  VCU_ESPTorqReqAvailability_Convert1 : DataTypeConversion  OutDataTypeStr=uint32
  VCU_ESPTorqReqAvailability_D : Product  Inputs=*/
  VCU_ESPTorqReqAvailability_F : Constant  OutDataTypeStr=single
  VCU_ESPTorqReqAvailability_L : simulink/Logic and Bit Operations/Bitwise Operator  logicop=AND  UseBitMask=on  BitMask=2  BitMaskRealWorld=Stored Integer
  VCU_ESPTorqReqAvailability_O : Constant  Value=0  OutDataTypeStr=single
  VCU_ESPTorqReqAvailability_S : ArithShift  BitShiftNumber=-1
  VCU_ESPTorqReqAvailability_sat : Saturate  UpperLimit=1  LowerLimit=0
  VCU_ESPTorqReqAvailability_st : Sum  Inputs=+-
  output1 : Outport
  output2 : Outport  Port=2
  output3 : Outport  Port=3
  output4 : Outport  Port=4
  output5 : Outport  Port=5
  output6 : Outport  Port=6
  output7 : Outport  Port=7
  output8 : Outport  Port=8
  wires:
  VCU_ESPTorqReqAvailability/1 -> VCU_ESPTorqReqAvailability_sat/1
  VCU_ESPTorqReqAvailability_sat/1 -> VCU_ESPTorqReqAvailability_st/1
  VCU_ESPTorqReqAvailability_O/1 -> VCU_ESPTorqReqAvailability_st/2
  VCU_ESPTorqReqAvailability_st/1 -> VCU_ESPTorqReqAvailability_D/1
  VCU_ESPTorqReqAvailability_F/1 -> VCU_ESPTorqReqAvailability_D/2
  VCU_ESPTorqReqAvailability_D/1 -> VCU_ESPTorqReqAvailabilityRon/1
  VCU_ESPTorqReqAvailabilityRon/1 -> VCU_ESPTorqReqAvailability_S/1
  VCU_ESPTorqReqAvailability_S/1 -> VCU_ESPTorqReqAvailability_1sat/1
  VCU_ESPTorqReqAvailability_1sat/1 -> VCU_ESPTorqReqAvailability_Convert1/1
  VCU_ESPTorqReqAvailability_Convert1/1 -> VCU_ESPTorqReqAvailability_L/1
  VCU_ESPTorqReqAvailability_L/1 -> VCU_ESPTorqReqAvailability_Convert/1
  VCU_ESPTorqReqAvailability_Convert/1 -> output7/1
  Constant1/1 -> output1/1
  Constant2/1 -> output2/1
  Constant3/1 -> output3/1
  Constant4/1 -> output4/1
  Constant5/1 -> output5/1
  Constant6/1 -> output6/1
  Constant8/1 -> output8/1

== system TxCAN3/TXMessage/VCU_EA/VCU_GearLevelPosSts ==
  VCU_GearLevelPosSts : Inport
  Constant{1..4,6..8} (7 alike) : Constant  Value=0  OutDataTypeStr=uint8
  VCU_GearLevelPosStsRon : Rounding  Operator=round
  VCU_GearLevelPosSts_1sat : Saturate  UpperLimit=3  LowerLimit=0
  VCU_GearLevelPosSts_Convert : DataTypeConversion  OutDataTypeStr=uint8
  VCU_GearLevelPosSts_Convert1 : DataTypeConversion  OutDataTypeStr=uint32
  VCU_GearLevelPosSts_D : Product  Inputs=*/
  VCU_GearLevelPosSts_F : Constant  OutDataTypeStr=single
  VCU_GearLevelPosSts_L : simulink/Logic and Bit Operations/Bitwise Operator  logicop=AND  UseBitMask=on  BitMask=3  BitMaskRealWorld=Stored Integer
  VCU_GearLevelPosSts_O : Constant  Value=0  OutDataTypeStr=single
  VCU_GearLevelPosSts_S : ArithShift
  VCU_GearLevelPosSts_sat : Saturate  UpperLimit=3  LowerLimit=0
  VCU_GearLevelPosSts_st : Sum  Inputs=+-
  output1 : Outport
  output2 : Outport  Port=2
  output3 : Outport  Port=3
  output4 : Outport  Port=4
  output5 : Outport  Port=5
  output6 : Outport  Port=6
  output7 : Outport  Port=7
  output8 : Outport  Port=8
  wires:
  VCU_GearLevelPosSts/1 -> VCU_GearLevelPosSts_sat/1
  VCU_GearLevelPosSts_sat/1 -> VCU_GearLevelPosSts_st/1
  VCU_GearLevelPosSts_O/1 -> VCU_GearLevelPosSts_st/2
  VCU_GearLevelPosSts_st/1 -> VCU_GearLevelPosSts_D/1
  VCU_GearLevelPosSts_F/1 -> VCU_GearLevelPosSts_D/2
  VCU_GearLevelPosSts_D/1 -> VCU_GearLevelPosStsRon/1
  VCU_GearLevelPosStsRon/1 -> VCU_GearLevelPosSts_S/1
  VCU_GearLevelPosSts_S/1 -> VCU_GearLevelPosSts_1sat/1
  VCU_GearLevelPosSts_1sat/1 -> VCU_GearLevelPosSts_Convert1/1
  VCU_GearLevelPosSts_Convert1/1 -> VCU_GearLevelPosSts_L/1
  VCU_GearLevelPosSts_L/1 -> VCU_GearLevelPosSts_Convert/1
  VCU_GearLevelPosSts_Convert/1 -> output5/1
  Constant1/1 -> output1/1
  Constant2/1 -> output2/1
  Constant3/1 -> output3/1
  Constant4/1 -> output4/1
  Constant6/1 -> output6/1
  Constant7/1 -> output7/1
  Constant8/1 -> output8/1

== system TxCAN3/TXMessage/VCU_EA/VCU_ParkingReqToEPB ==
  VCU_ParkingReqToEPB : Inport
  Constant{1..6,8} (7 alike) : Constant  Value=0  OutDataTypeStr=uint8
  VCU_ParkingReqToEPBRon : Rounding  Operator=round
  VCU_ParkingReqToEPB_1sat : Saturate  UpperLimit=12  LowerLimit=0
  VCU_ParkingReqToEPB_Convert : DataTypeConversion  OutDataTypeStr=uint8
  VCU_ParkingReqToEPB_Convert1 : DataTypeConversion  OutDataTypeStr=uint32
  VCU_ParkingReqToEPB_D : Product  Inputs=*/
  VCU_ParkingReqToEPB_F : Constant  OutDataTypeStr=single
  VCU_ParkingReqToEPB_L : simulink/Logic and Bit Operations/Bitwise Operator  logicop=AND  UseBitMask=on  BitMask=12  BitMaskRealWorld=Stored Integer
  VCU_ParkingReqToEPB_O : Constant  Value=0  OutDataTypeStr=single
  VCU_ParkingReqToEPB_S : ArithShift  BitShiftNumber=-2
  VCU_ParkingReqToEPB_sat : Saturate  UpperLimit=3  LowerLimit=0
  VCU_ParkingReqToEPB_st : Sum  Inputs=+-
  output1 : Outport
  output2 : Outport  Port=2
  output3 : Outport  Port=3
  output4 : Outport  Port=4
  output5 : Outport  Port=5
  output6 : Outport  Port=6
  output7 : Outport  Port=7
  output8 : Outport  Port=8
  wires:
  VCU_ParkingReqToEPB/1 -> VCU_ParkingReqToEPB_sat/1
  VCU_ParkingReqToEPB_sat/1 -> VCU_ParkingReqToEPB_st/1
  VCU_ParkingReqToEPB_O/1 -> VCU_ParkingReqToEPB_st/2
  VCU_ParkingReqToEPB_st/1 -> VCU_ParkingReqToEPB_D/1
  VCU_ParkingReqToEPB_F/1 -> VCU_ParkingReqToEPB_D/2
  VCU_ParkingReqToEPB_D/1 -> VCU_ParkingReqToEPBRon/1
  VCU_ParkingReqToEPBRon/1 -> VCU_ParkingReqToEPB_S/1
  VCU_ParkingReqToEPB_S/1 -> VCU_ParkingReqToEPB_1sat/1
  VCU_ParkingReqToEPB_1sat/1 -> VCU_ParkingReqToEPB_Convert1/1
  VCU_ParkingReqToEPB_Convert1/1 -> VCU_ParkingReqToEPB_L/1
  VCU_ParkingReqToEPB_L/1 -> VCU_ParkingReqToEPB_Convert/1
  VCU_ParkingReqToEPB_Convert/1 -> output7/1
  Constant1/1 -> output1/1
  Constant2/1 -> output2/1
  Constant3/1 -> output3/1
  Constant4/1 -> output4/1
  Constant5/1 -> output5/1
  Constant6/1 -> output6/1
  Constant8/1 -> output8/1

== system TxCAN3/TXMessage/VCU_EA/VCU_RollingCounter ==
  VCU_RollingCounter : Inport
  Constant{1..6,8} (7 alike) : Constant  Value=0  OutDataTypeStr=uint8
  VCU_RollingCounterRon : Rounding  Operator=round
  VCU_RollingCounter_1sat : Saturate  UpperLimit=240  LowerLimit=0
  VCU_RollingCounter_Convert : DataTypeConversion  OutDataTypeStr=uint8
  VCU_RollingCounter_Convert1 : DataTypeConversion  OutDataTypeStr=uint32
  VCU_RollingCounter_D : Product  Inputs=*/
  VCU_RollingCounter_F : Constant  OutDataTypeStr=single
  VCU_RollingCounter_L : simulink/Logic and Bit Operations/Bitwise Operator  logicop=AND  UseBitMask=on  BitMask=240  BitMaskRealWorld=Stored Integer
  VCU_RollingCounter_O : Constant  Value=0  OutDataTypeStr=single
  VCU_RollingCounter_S : ArithShift  BitShiftNumber=-4
  VCU_RollingCounter_sat : Saturate  UpperLimit=15  LowerLimit=0
  VCU_RollingCounter_st : Sum  Inputs=+-
  output1 : Outport
  output2 : Outport  Port=2
  output3 : Outport  Port=3
  output4 : Outport  Port=4
  output5 : Outport  Port=5
  output6 : Outport  Port=6
  output7 : Outport  Port=7
  output8 : Outport  Port=8
  wires:
  VCU_RollingCounter/1 -> VCU_RollingCounter_sat/1
  VCU_RollingCounter_sat/1 -> VCU_RollingCounter_st/1
  VCU_RollingCounter_O/1 -> VCU_RollingCounter_st/2
  VCU_RollingCounter_st/1 -> VCU_RollingCounter_D/1
  VCU_RollingCounter_F/1 -> VCU_RollingCounter_D/2
  VCU_RollingCounter_D/1 -> VCU_RollingCounterRon/1
  VCU_RollingCounterRon/1 -> VCU_RollingCounter_S/1
  VCU_RollingCounter_S/1 -> VCU_RollingCounter_1sat/1
  VCU_RollingCounter_1sat/1 -> VCU_RollingCounter_Convert1/1
  VCU_RollingCounter_Convert1/1 -> VCU_RollingCounter_L/1
  VCU_RollingCounter_L/1 -> VCU_RollingCounter_Convert/1
  VCU_RollingCounter_Convert/1 -> output7/1
  Constant1/1 -> output1/1
  Constant2/1 -> output2/1
  Constant3/1 -> output3/1
  Constant4/1 -> output4/1
  Constant5/1 -> output5/1
  Constant6/1 -> output6/1
  Constant8/1 -> output8/1

== system TxCAN3/TXMessage/VCU_EA/VCU_VehicleSts ==
  VCU_VehicleSts : Inport
  Constant{1..4,6..8} (7 alike) : Constant  Value=0  OutDataTypeStr=uint8
  VCU_VehicleStsRon : Rounding  Operator=round
  VCU_VehicleSts_1sat : Saturate  UpperLimit=4  LowerLimit=0
  VCU_VehicleSts_Convert : DataTypeConversion  OutDataTypeStr=uint8
  VCU_VehicleSts_Convert1 : DataTypeConversion  OutDataTypeStr=uint32
  VCU_VehicleSts_D : Product  Inputs=*/
  VCU_VehicleSts_F : Constant  OutDataTypeStr=single
  VCU_VehicleSts_L : simulink/Logic and Bit Operations/Bitwise Operator  logicop=AND  UseBitMask=on  BitMask=4  BitMaskRealWorld=Stored Integer
  VCU_VehicleSts_O : Constant  Value=0  OutDataTypeStr=single
  VCU_VehicleSts_S : ArithShift  BitShiftNumber=-2
  VCU_VehicleSts_sat : Saturate  UpperLimit=1  LowerLimit=0
  VCU_VehicleSts_st : Sum  Inputs=+-
  output1 : Outport
  output2 : Outport  Port=2
  output3 : Outport  Port=3
  output4 : Outport  Port=4
  output5 : Outport  Port=5
  output6 : Outport  Port=6
  output7 : Outport  Port=7
  output8 : Outport  Port=8
  wires:
  VCU_VehicleSts/1 -> VCU_VehicleSts_sat/1
  VCU_VehicleSts_sat/1 -> VCU_VehicleSts_st/1
  VCU_VehicleSts_O/1 -> VCU_VehicleSts_st/2
  VCU_VehicleSts_st/1 -> VCU_VehicleSts_D/1
  VCU_VehicleSts_F/1 -> VCU_VehicleSts_D/2
  VCU_VehicleSts_D/1 -> VCU_VehicleStsRon/1
  VCU_VehicleStsRon/1 -> VCU_VehicleSts_S/1
  VCU_VehicleSts_S/1 -> VCU_VehicleSts_1sat/1
  VCU_VehicleSts_1sat/1 -> VCU_VehicleSts_Convert1/1
  VCU_VehicleSts_Convert1/1 -> VCU_VehicleSts_L/1
  VCU_VehicleSts_L/1 -> VCU_VehicleSts_Convert/1
  VCU_VehicleSts_Convert/1 -> output5/1
  Constant1/1 -> output1/1
  Constant2/1 -> output2/1
  Constant3/1 -> output3/1
  Constant4/1 -> output4/1
  Constant6/1 -> output6/1
  Constant7/1 -> output7/1
  Constant8/1 -> output8/1

== system TxCAN3/TXMessage/VCU_EA/VCU_Vehicle_Warning ==
  VCU_Vehicle_Warning : Inport
  Constant{1..3,5..8} (7 alike) : Constant  Value=0  OutDataTypeStr=uint8
  VCU_Vehicle_WarningRon : Rounding  Operator=round
  VCU_Vehicle_Warning_1sat : Saturate  UpperLimit=192  LowerLimit=0
  VCU_Vehicle_Warning_Convert : DataTypeConversion  OutDataTypeStr=uint8
  VCU_Vehicle_Warning_Convert1 : DataTypeConversion  OutDataTypeStr=uint32
  VCU_Vehicle_Warning_D : Product  Inputs=*/
  VCU_Vehicle_Warning_F : Constant  OutDataTypeStr=single
  VCU_Vehicle_Warning_L : simulink/Logic and Bit Operations/Bitwise Operator  logicop=AND  UseBitMask=on  BitMask=192  BitMaskRealWorld=Stored Integer
  VCU_Vehicle_Warning_O : Constant  Value=0  OutDataTypeStr=single
  VCU_Vehicle_Warning_S : ArithShift  BitShiftNumber=-6
  VCU_Vehicle_Warning_sat : Saturate  UpperLimit=3  LowerLimit=0
  VCU_Vehicle_Warning_st : Sum  Inputs=+-
  output1 : Outport
  output2 : Outport  Port=2
  output3 : Outport  Port=3
  output4 : Outport  Port=4
  output5 : Outport  Port=5
  output6 : Outport  Port=6
  output7 : Outport  Port=7
  output8 : Outport  Port=8
  wires:
  VCU_Vehicle_Warning/1 -> VCU_Vehicle_Warning_sat/1
  VCU_Vehicle_Warning_sat/1 -> VCU_Vehicle_Warning_st/1
  VCU_Vehicle_Warning_O/1 -> VCU_Vehicle_Warning_st/2
  VCU_Vehicle_Warning_st/1 -> VCU_Vehicle_Warning_D/1
  VCU_Vehicle_Warning_F/1 -> VCU_Vehicle_Warning_D/2
  VCU_Vehicle_Warning_D/1 -> VCU_Vehicle_WarningRon/1
  VCU_Vehicle_WarningRon/1 -> VCU_Vehicle_Warning_S/1
  VCU_Vehicle_Warning_S/1 -> VCU_Vehicle_Warning_1sat/1
  VCU_Vehicle_Warning_1sat/1 -> VCU_Vehicle_Warning_Convert1/1
  VCU_Vehicle_Warning_Convert1/1 -> VCU_Vehicle_Warning_L/1
  VCU_Vehicle_Warning_L/1 -> VCU_Vehicle_Warning_Convert/1
  VCU_Vehicle_Warning_Convert/1 -> output4/1
  Constant1/1 -> output1/1
  Constant2/1 -> output2/1
  Constant3/1 -> output3/1
  Constant5/1 -> output5/1
  Constant6/1 -> output6/1
  Constant7/1 -> output7/1
  Constant8/1 -> output8/1
